simulink model "TF_SISO_orig_test"  (Simulink 7.5)
settings: Solver=ode45  StartTime=0.0  StopTime=10000  RelTol=1e-3
undefined symbols (not defined in the file or in its folder): init_cond, Ts
libraries: simulink x5
settings Model: Creator=laszlodobos  LastModifiedBy=laszlodobos  ExtModeAutoUpdateStatusClock=off
settings DataIOCC: SaveFinalState=on
settings OptimizationCC: InitFltsAndDblsToZero=on
settings DebuggingCC: SaveWithParameterizedLinksMsg=none  StrictBusMsg=Warning
settings GRTTargetCC: TargetFcnLib=ansi_tfl_tmw.mat

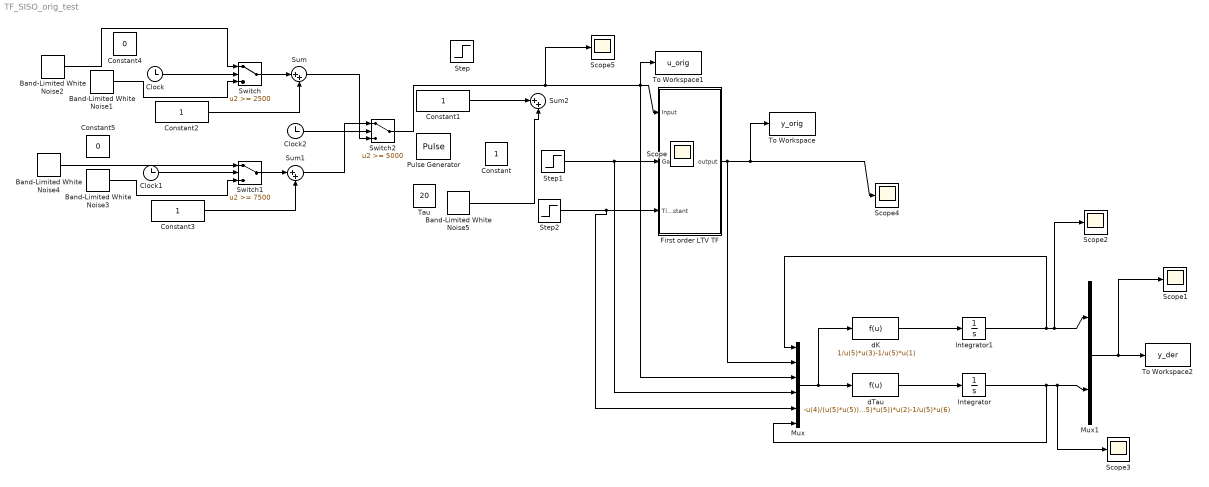
== system TF_SISO_orig_test ==
  Band-Limited White Noise1 : simulink/Sources/Band-Limited White Noise  SystemSampleTime=-1  Cov=[1]  Ts=8  seed=0
  Band-Limited White Noise2 : simulink/Sources/Band-Limited White Noise  SystemSampleTime=-1  Cov=[1]  Ts=60  seed=0
  Band-Limited White Noise3 : simulink/Sources/Band-Limited White Noise  SystemSampleTime=-1  Cov=[0.1]  Ts=6  seed=0
  Band-Limited White Noise4 : simulink/Sources/Band-Limited White Noise  SystemSampleTime=-1  Cov=[1]  Ts=30  seed=0
  Band-Limited White Noise5 : simulink/Sources/Band-Limited White Noise  SystemSampleTime=-1  Cov=[1]  Ts=60  seed=0
  Clock : Clock
      settings: Decimation=10
  Clock1 : Clock
      settings: Decimation=10
  Clock2 : Clock
      settings: Decimation=10
  Constant{,1..3} (4 alike) : Constant  OutDataType=sfix(16)  OutScaling=2^0
  Constant4 : Constant  Value=0  OutDataType=sfix(16)  OutScaling=2^0
  Constant5 : Constant  Value=0  OutDataType=sfix(16)  OutScaling=2^0
  First order LTV TF : Subsystem  mask{Initial=init_cond}
      mask prompts: Initial "Initial Condition"
  Integrator : Integrator
  Integrator1 : Integrator
  Mux : Mux  Inputs=6
  Mux1 : Mux  Inputs=2
  Pulse Generator : DiscretePulseGenerator  PulseType=Time based  Amplitude=1  Period=10  PulseWidth=50  PhaseDelay=0  SampleTime=1
  Scope{,1..5} (6 alike) : Scope
      Scope settings: YMin=0.975  YMax=1.045
      Scope2 settings: SaveName=ScopeData2
      Scope3 settings: SaveName=ScopeData3
      Scope4 settings: SaveName=ScopeData4
      Scope5 settings: SaveName=ScopeData5
  Step : Step  Time=300  Before=1  After=2  SampleTime=Ts
  Step1 : Step  Time=500  Before=1  SampleTime=Ts
  Step2 : Step  Time=400  Before=10  After=10  SampleTime=Ts
  Sum : Sum  Inputs=|++  OutDataType=sfix(16)  OutScaling=2^0
  Sum1 : Sum  Inputs=|++  OutDataType=sfix(16)  OutScaling=2^0
  Sum2 : Sum  Inputs=|++  OutDataType=sfix(16)  OutScaling=2^0
  Switch : Switch  Threshold=2500
  Switch1 : Switch  Threshold=7500
  Switch2 : Switch  Threshold=5000
  Tau : Constant  Value=20  OutDataType=sfix(16)  OutScaling=2^0
  To Workspace : ToWorkspace  VariableName=y_orig  SampleTime=Ts  SaveFormat=Structure With Time
  To Workspace1 : ToWorkspace  VariableName=u_orig  SampleTime=Ts  SaveFormat=Structure With Time
  To Workspace2 : ToWorkspace  VariableName=y_der  SampleTime=Ts  SaveFormat=Array
  dK : Fcn  Expr=1/u(5)*u(3)-1/u(5)*u(1)
  dTau : Fcn  Expr=-u(4)/(u(5)*u(5))*u(3)+1/(u(5)*u(5))*u(2)-1/u(5)*u(6)
  wires:
  Step1/1 -> First order LTV TF/2(Gain), Mux/4
  Step2/1 -> First order LTV TF/3(Time constant), Mux/5
  First order LTV TF/1(output) -> Scope/1, To Workspace/1, Scope4/1, Mux/2
  Integrator/1 -> Mux/6, Mux1/2, Scope3/1
  Mux/1 -> dTau/1, dK/1
  dTau/1 -> Integrator/1
  Integrator1/1 -> Mux/1, Mux1/1, Scope2/1
  dK/1 -> Integrator1/1
  Mux1/1 -> To Workspace2/1, Scope1/1
  Constant2/1 -> Sum/2
  Clock/1 -> Switch/2
  Switch/1 -> Sum/1
  Constant3/1 -> Sum1/2
  Clock1/1 -> Switch1/2
  Switch1/1 -> Sum1/1
  Clock2/1 -> Switch2/2
  Sum1/1 -> Switch2/1
  Band-Limited White Noise2/1 -> Switch/1
  Band-Limited White Noise4/1 -> Switch1/1
  Band-Limited White Noise1/1 -> Switch/3
  Band-Limited White Noise3/1 -> Switch1/3
  Sum/1 -> Switch2/3
  Constant1/1 -> Sum2/1
  Band-Limited White Noise5/1 -> Sum2/2
  Switch2/1 -> Scope5/1, First order LTV TF/1(Input), To Workspace1/1, Mux/3

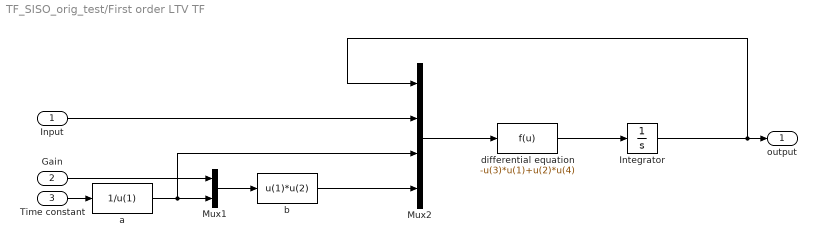
== system TF_SISO_orig_test/First order LTV TF ==
  Input : Inport  OutDataType=sfix(16)  OutScaling=2^0
  Gain : Inport  Port=2  OutDataType=sfix(16)  OutScaling=2^0
  Time constant : Inport  Port=3  OutDataType=sfix(16)  OutScaling=2^0
  Integrator : Integrator  InitialCondition=Initial
  Mux1 : Mux  Inputs=2
  Mux2 : Mux
  a : Fcn  Expr=1/u(1)
  b : Fcn  Expr=u(1)*u(2)
  differential equation : Fcn  Expr=-u(3)*u(1)+u(2)*u(4)
  output : Outport  OutDataType=sfix(16)  OutScaling=2^0
  wires:
  Integrator/1 -> Mux2/1, output/1
  differential equation/1 -> Integrator/1
  Mux2/1 -> differential equation/1
  b/1 -> Mux2/4
  Mux1/1 -> b/1
  a/1 -> Mux1/2, Mux2/3
  Input/1 -> Mux2/2
  Gain/1 -> Mux1/1
  Time constant/1 -> a/1
